simulink model "sml_braitenberg"  (R2016a)
settings: Solver=VariableStepAuto  StartTime=0.0  StopTime=150  RelTol=1e-3
libraries: simulink x1
settings Model: Creator=Duy Nam  LastModifiedBy=Duy Nam

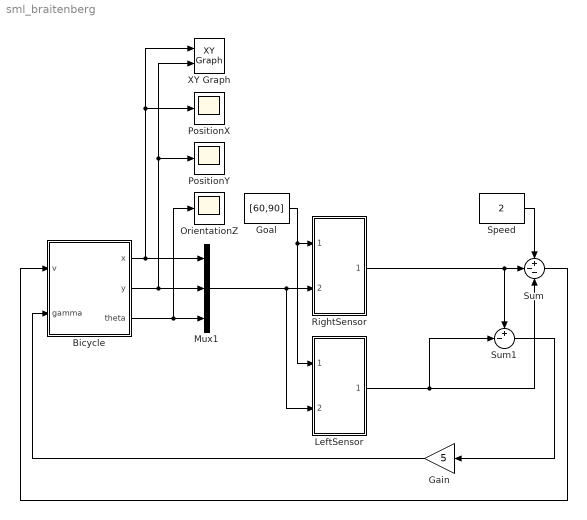
== system sml_braitenberg ==
  Bicycle : Subsystem
  Gain : Gain  Gain=5
  Goal : Constant  Value=[60,90]
  LeftSensor : Subsystem
  Mux1 : Mux  Inputs=3
  OrientationZ : Scope
  PositionX : Scope
  PositionY : Scope
  RightSensor : Subsystem
  Speed : Constant  Value=2
  Sum : Sum  Inputs=+--
  Sum1 : Sum  Inputs=+-|
  XY Graph : simulink/Sinks/XY Graph  xmin=0  xmax=100  ymin=0  ymax=100  st=-1
  wires:
  Bicycle/1(x) -> PositionX/1, XY Graph/1, Mux1/1
  Bicycle/3(theta) -> OrientationZ/1, Mux1/3
  Bicycle/2(y) -> Mux1/2, PositionY/1, XY Graph/2
  Speed/1 -> Sum/1
  Sum/1 -> Bicycle/1(v)
  Goal/1 -> LeftSensor/1(goal), RightSensor/1(goal)
  Mux1/1 -> LeftSensor/2(robot_pose), RightSensor/2(robot_pose)
  Sum1/1 -> Gain/1
  Gain/1 -> Bicycle/2(gamma)
  RightSensor/1(sensor) -> Sum1/1, Sum/2
  LeftSensor/1(sensor) -> Sum/3, Sum1/2

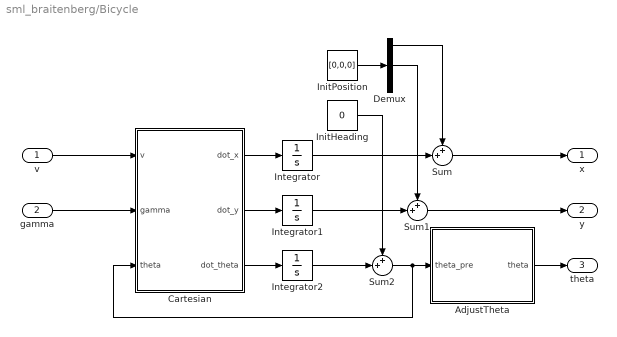
== system sml_braitenberg/Bicycle ==
  v : Inport
  gamma : Inport  Port=2
  AdjustTheta : MATLAB Function  TreatAsAtomicUnit=on
  Cartesian : MATLAB Function  TreatAsAtomicUnit=on
  Demux : Demux  Outputs=3
  InitHeading : Constant  Value=0
  InitPosition : Constant  Value=[0,0,0]
  Integrator : Integrator
  Integrator1 : Integrator
  Integrator2 : Integrator
  Sum : Sum  Inputs=++|
  Sum1 : Sum  Inputs=++|
  Sum2 : Sum  Inputs=++|
  x : Outport
  y : Outport  Port=2
  theta : Outport  Port=3
  wires:
  Cartesian/1(dot_x) -> Integrator/1
  Integrator/1 -> Sum/2
  Cartesian/2(dot_y) -> Integrator1/1
  Integrator1/1 -> Sum1/2
  Cartesian/3(dot_theta) -> Integrator2/1
  AdjustTheta/1(theta) -> theta/1
  Sum2/1 -> Cartesian/3(theta), AdjustTheta/1(theta_pre)
  v/1 -> Cartesian/1(v)
  gamma/1 -> Cartesian/2(gamma)
  InitPosition/1 -> Demux/1
  Sum/1 -> x/1
  Demux/1 -> Sum/1
  Sum1/1 -> y/1
  Demux/2 -> Sum1/1
  Integrator2/1 -> Sum2/2
  InitHeading/1 -> Sum2/1

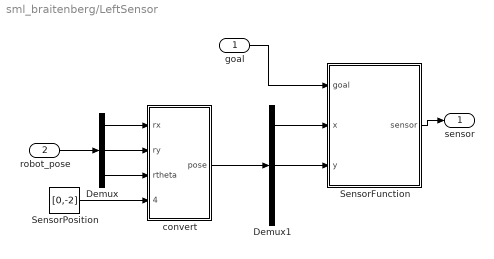
== system sml_braitenberg/LeftSensor ==
  goal : Inport
  robot_pose : Inport  Port=2
  Demux : Demux  Outputs=3
  Demux1 : Demux  Outputs=3
  SensorFunction : MATLAB Function  TreatAsAtomicUnit=on
  SensorPosition : Constant  Value=[0,-2]
  convert : MATLAB Function  TreatAsAtomicUnit=on
  sensor : Outport
  wires:
  Demux1/2 -> SensorFunction/3(y)
  Demux1/1 -> SensorFunction/2(x)
  Demux/3 -> convert/3(rtheta)
  Demux/2 -> convert/2(ry)
  Demux/1 -> convert/1(rx)
  goal/1 -> SensorFunction/1(goal)
  SensorPosition/1 -> convert/4(sensor_pose)
  convert/1(pose) -> Demux1/1
  robot_pose/1 -> Demux/1
  SensorFunction/1(sensor) -> sensor/1

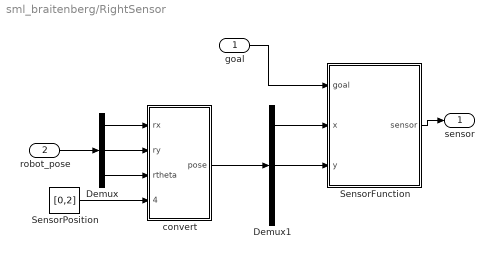
== system sml_braitenberg/RightSensor ==
  goal : Inport
  robot_pose : Inport  Port=2
  Demux : Demux  Outputs=3
  Demux1 : Demux  Outputs=3
  SensorFunction : MATLAB Function  TreatAsAtomicUnit=on
  SensorPosition : Constant  Value=[0,2]
  convert : MATLAB Function  TreatAsAtomicUnit=on
  sensor : Outport
  wires:
  SensorFunction/1(sensor) -> sensor/1
  robot_pose/1 -> Demux/1
  convert/1(pose) -> Demux1/1
  SensorPosition/1 -> convert/4(sensor_pose)
  goal/1 -> SensorFunction/1(goal)
  Demux/1 -> convert/1(rx)
  Demux/2 -> convert/2(ry)
  Demux/3 -> convert/3(rtheta)
  Demux1/1 -> SensorFunction/2(x)
  Demux1/2 -> SensorFunction/3(y)

== matlab function sml_braitenberg/Bicycle/AdjustTheta ==
  data: theta_pre input; theta output
function theta = AdjustTheta(theta_pre)
% ADJUSTTHETA Adjust the heading angle always between [-pi/2;pi/2]
%% INPUTS
% theta_pre = The heading angle before adjust
%% OUTPUTS
% theta = The heading angle after adjust
%% AdjustTheta
theta = theta_pre - 2*pi*floor((theta_pre + pi)/(2*pi));
end

== matlab function sml_braitenberg/Bicycle/Cartesian ==
  data: dot_x output; dot_y output; v input; gamma input; theta input; dot_theta output
function [dot_x, dot_y, dot_theta] = Cartesian(v, gamma, theta)
% CARTESIAN Compute the velocity of robot in world frame
%% INPUTS
% v     = The velocity of the back wheel
% gamma = The steering wheel angle
% theta = The heading angle
%% OUTPUTS
% dot_x     = The velocity of robot in world frame x-axis
% dot_y     = The velocity of robot in world frame y-axis
% dot theta = The rate of change of heading
%% PARAMETERS
L = params_bicycle();
%% Cartesian
dot_x = v*cos(theta);
dot_y = v*sin(theta);
dot_theta = v/L*tan(gamma);
end

== matlab function sml_braitenberg/RightSensor/SensorFunction ==
  data: goal input; sensor output; x input; y input
function sensor = SensorFunction(goal, x, y)
% SENSORFUNCTION Return value of sensor
%% INPUTS
% goal  = The goal position in world frame
% x     = The sensor position x in world frame
% y     = The sensor position y in world frame
%% OUTPUTS
% sensor = The value get from sensor
%% Assign values
gx = goal(1);
gy = goal(2);
%% Sense
sensor = 200/((x-gx)^2 + (y-gy)^2 + 200);
end

== matlab function sml_braitenberg/RightSensor/convert ==
  data: rx input; ry input; pose output; rtheta input; sensor_pose input
function pose = convert(rx, ry, rtheta, sensor_pose)
% CONVERT convert to position of sensor in the world frame
%% INPUTS
% rx            = The position x of robot in the world frame
% ry            = The position y of robot in the world frame
% rtheta        = The orientation z of robot in the world frame
% sensor_pose   = The position of sensor relate with robot
%% OUTPUT
% pose = The position of sensor in the world frame
%% Assign values
dx = sensor_pose(1);
dy = sensor_pose(2);
%% Create the robot pose matrix
T = [cos(rtheta) -sin(rtheta) rx;...
     sin(rtheta) cos(rtheta) ry;...
     0 0 1];
%% Compute the sensor pose
pose = T*[dx;dy;1];
end

== matlab function sml_braitenberg/LeftSensor/SensorFunction ==
  data: goal input; sensor output; x input; y input
function sensor = SensorFunction(goal, x, y)
% SENSORFUNCTION Return value of sensor
%% INPUTS
% goal  = The goal position in world frame
% x     = The sensor position x in world frame
% y     = The sensor position y in world frame
%% OUTPUTS
% sensor = The value get from sensor
%% Assign values
gx = goal(1);
gy = goal(2);
%% Sense
sensor = 200/((x-gx)^2 + (y-gy)^2 + 200);
end

== matlab function sml_braitenberg/LeftSensor/convert ==
  data: rx input; ry input; pose output; rtheta input; sensor_pose input
function pose = convert(rx, ry, rtheta, sensor_pose)
% CONVERT convert to position of sensor in the world frame
%% INPUTS
% rx            = The position x of robot in the world frame
% ry            = The position y of robot in the world frame
% rtheta        = The orientation z of robot in the world frame
% sensor_pose   = The position of sensor relate with robot
%% OUTPUT
% pose = The position of sensor in the world frame
%% Assign values
dx = sensor_pose(1);
dy = sensor_pose(2);
%% Create the robot pose matrix
T = [cos(rtheta) -sin(rtheta) rx;...
     sin(rtheta) cos(rtheta) ry;...
     0 0 1];
%% Compute the sensor pose
pose = T*[dx;dy;1];
end
